simulink model "NCO"  (R2024b)
settings: Solver=FixedStepDiscrete  StartTime=0.0  StopTime=sysParams.FPGAClkPeriod*1e4  RelTol=1e-3
PreLoadFcn:
  | init;
StopFcn:
  | run("NCOmetrics");
undefined symbols (not defined in the file): iChain, sysParams, tuningWord
libraries: dsphdlsigops2 x2
settings Model: DataTypeOverride=Off  Creator=aless  LastModifiedBy=aless
settings SolverCC: PositivePriorityOrder=on
settings OptimizationCC: BlockReduction=off  ConditionallyExecuteInputs=off  DefaultParameterBehavior=Inlined  InheritOutputTypeSmallerThanSingle=on  EnhancedBackFolding=on  PassReuseOutputArgsAs=Individual arguments  ZeroExternalMemoryAtStartup=off  ZeroInternalMemoryAtStartup=off  MaxStackSize=64  OptimizeBlockOrder=speed  DifferentSizesBufferReuse=on  OptimizationCustomize=off  EfficientTunableParamExpr=on
settings DebuggingCC: AlgebraicLoopMsg=error  SingleTaskRateTransMsg=error  ParameterTunabilityLossMsg=error  UnconnectedInputMsg=warning  UnconnectedOutputMsg=warning  UnconnectedLineMsg=warning
settings HardwareCC: ProdBitPerPointer=32  ProdBitPerSizeT=32  ProdBitPerPtrDiffT=32  ProdLargestAtomicFloat=None  ProdIntDivRoundTo=Undefined  ProdEndianess=Unspecified  ProdWordSize=32  ProdHWDeviceType=ASIC/FPGA->ASIC/FPGA  TargetBitPerPointer=64  TargetBitPerSizeT=64  TargetBitPerPtrDiffT=64  TargetLongLongMode=on  TargetIntDivRoundTo=Zero  TargetEndianess=LittleEndian  TargetWordSize=64  TargetHWDeviceType=Custom Processor->MATLAB Host Computer  ProdEqTarget=off  HardwareBoardFeatureSet=SoCBlockset
settings ModelReferenceCC: ModelReferenceNumInstancesAllowed=Single
settings RTWCC: Description=Embedded Coder  SystemTargetFile=ert.tlc  HardwareBoard=Xilinx Zynq UltraScale+ RFSoC ZCU208 Evaluation Kit  TLCOptions="-aInlineSetEventsForThisBaseRateFcn=TLC_FALSE -aSuppressMultiTaskScheduler=TLC_FALSE  -aRateBasedStepFcn=0"  TemplateMakefile=ert_default_tmf  Toolchain=Linaro AArch64 Linux v6.3.1
settings CodeAppCC: ForceParamTrailComments=on  IgnoreCustomStorageClasses=off  OperatorAnnotations=on  SimulinkDataObjDesc=on  SFDataObjDesc=on  InsertBlockDesc=on

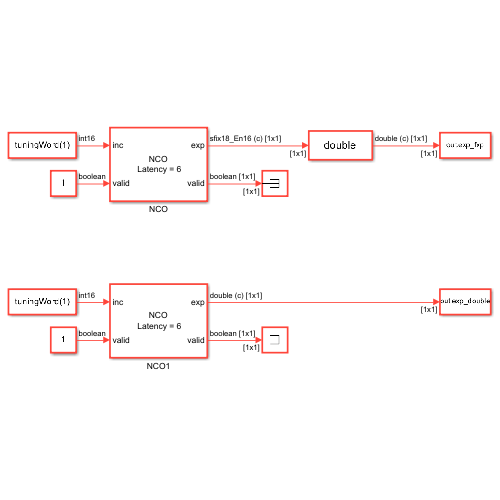
[thumbnail: Simulink's stored preview of the top-level diagram]
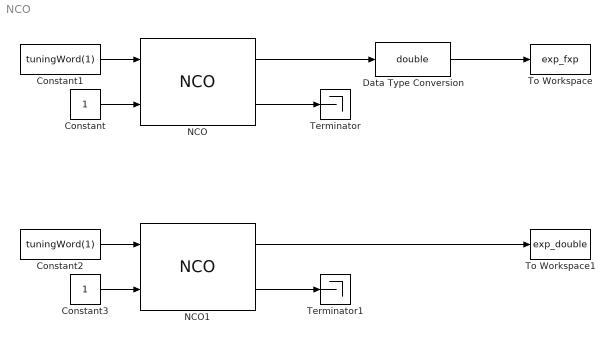
== system NCO ==
  Constant : Constant  OutDataTypeStr=boolean  SampleTime=sysParams.FPGAClkPeriod/iChain.interpFactor
  Constant1 : Constant  Value=tuningWord(1)  OutDataTypeStr=fixdt(1,FXP.NCOphaseAccWL,0)  SampleTime=sysParams.FPGAClkPeriod/iChain.interpFactor
  Constant2 : Constant  Value=tuningWord(1)  OutDataTypeStr=fixdt(1,FXP.NCOphaseAccWL,0)  SampleTime=sysParams.FPGAClkPeriod/iChain.interpFactor
  Constant3 : Constant  OutDataTypeStr=boolean  SampleTime=sysParams.FPGAClkPeriod/iChain.interpFactor
  Data Type Conversion : DataTypeConversion  OutDataTypeStr=double  SaturateOnIntegerOverflow=off  RndMeth=Floor
  NCO : dsphdlsigops2/NCO  PhaseIncrementSource=Input port  PhaseIncrement=100  PhaseOffsetSource=Property  PhaseOffset=0  DitherSource=None  NumDitherBits=4  SamplesPerFrame=1  LUTCompress=on  ResetAction=off  Waveform=Complex exponential  PhasePort=off  SimulateUsing=Code generation  AccumulatorWL=FXP.NCOphaseAccWL  PhaseQuantization=on  NumQuantizerAccumulatorBits=FXP.NCOlutAddressWL  OutputDataType=Binary point scaling  OutputWL=FXP.sampWL  OutputFL=FXP.sampFL
  NCO1 : dsphdlsigops2/NCO  PhaseIncrementSource=Input port  PhaseIncrement=100  PhaseOffsetSource=Property  PhaseOffset=0  DitherSource=None  NumDitherBits=4  SamplesPerFrame=1  LUTCompress=off  ResetAction=off  Waveform=Complex exponential  PhasePort=off  SimulateUsing=Code generation  AccumulatorWL=FXP.NCOphaseAccWL  PhaseQuantization=off  NumQuantizerAccumulatorBits=FXP.NCOlutAddressWL  OutputDataType=double  OutputWL=FXP.sampWL  OutputFL=FXP.sampFL
  Terminator : Terminator
  Terminator1 : Terminator
  To Workspace : ToWorkspace  VariableName=exp_fxp  SampleTime=-1
      settings: Save2DSignal=2-D array (concatenate along first dimension)
  To Workspace1 : ToWorkspace  VariableName=exp_double  SampleTime=-1
      settings: Save2DSignal=2-D array (concatenate along first dimension)
  wires:
  Constant/1 -> NCO/2
  NCO/2 -> Terminator/1
  Constant1/1 -> NCO/1
  NCO/1 -> Data Type Conversion/1
  Data Type Conversion/1 -> To Workspace/1
  NCO1/1 -> To Workspace1/1
  Constant2/1 -> NCO1/1
  Constant3/1 -> NCO1/2
  NCO1/2 -> Terminator1/1
